simulink model "lab1"  (R2020a)
settings: Solver=VariableStepAuto  StartTime=0.0  StopTime=100  RelTol=1e-3
settings Model: Creator=L1.3-21_2  LastModifiedBy=admin
settings DataIOCC: ReturnWorkspaceOutputs=off
settings DebuggingCC: ArithmeticOperatorsInVariantConditions=warning
settings SFSimCC: SimUseLocalCustomCode=off  CustomCodeUndefinedFunction=UseInterfaceOnly
settings RTWCC: RTWUseLocalCustomCode=off

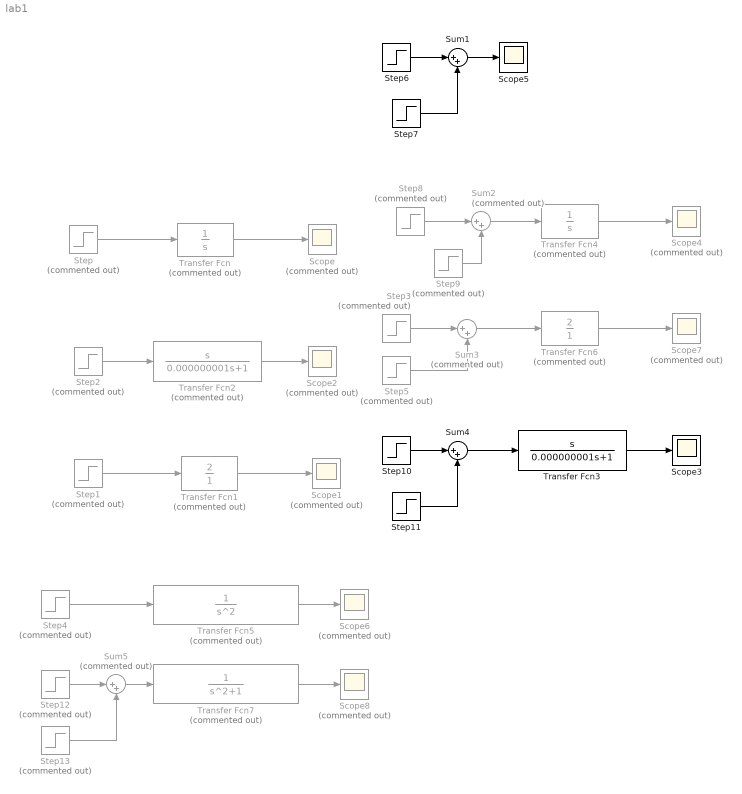
== system lab1 ==
  Scope{,1..2,4,6..8} (7 alike) : Scope  Commented=on
  Scope3 : Scope
  Scope5 : Scope
  Step{,1..2,4} (4 alike) : Step  Commented=on  SampleTime=0
  Step10 : Step  After=100000  SampleTime=0
  Step11 : Step  Time=1.0001  After=-100000  SampleTime=0
  Step12 : Step  Commented=on  After=100000  SampleTime=0
  Step13 : Step  Commented=on  Time=1.0001  After=-100000  SampleTime=0
  Step3 : Step  Commented=on  After=100000  SampleTime=0
  Step5 : Step  Commented=on  Time=1.00001  After=-100000  SampleTime=0
  Step6 : Step  After=100000  SampleTime=0
  Step7 : Step  Time=1.0001  After=-100000  SampleTime=0
  Step8 : Step  Commented=on  After=100000  SampleTime=0
  Step9 : Step  Commented=on  Time=1.00001  After=-100000  SampleTime=0
  Sum1 : Sum  Inputs=|++
  Sum2 : Sum  Commented=on  Inputs=|++
  Sum3 : Sum  Commented=on  Inputs=|++
  Sum4 : Sum  Inputs=|++
  Sum5 : Sum  Commented=on  Inputs=|++
  Transfer Fcn : TransferFcn  Commented=on  Denominator=[1 0]
  Transfer Fcn1 : TransferFcn  Commented=on  Numerator=[2]  Denominator=[1]
  Transfer Fcn2 : TransferFcn  Commented=on  Numerator=[1 0]  Denominator=[0.000000001 1]
  Transfer Fcn3 : TransferFcn  Numerator=[1 0]  Denominator=[0.000000001 1]
  Transfer Fcn4 : TransferFcn  Commented=on  Denominator=[1 0]
  Transfer Fcn5 : TransferFcn  Commented=on  Denominator=[1 0 0]
  Transfer Fcn6 : TransferFcn  Commented=on  Numerator=[2]  Denominator=[1]
  Transfer Fcn7 : TransferFcn  Commented=on  Denominator=[1 0 1]
  wires:
  Step/1 -> Transfer Fcn/1
  Transfer Fcn/1 -> Scope/1
  Transfer Fcn1/1 -> Scope1/1
  Step1/1 -> Transfer Fcn1/1
  Transfer Fcn2/1 -> Scope2/1
  Step2/1 -> Transfer Fcn2/1
  Transfer Fcn4/1 -> Scope4/1
  Step6/1 -> Sum1/1
  Step7/1 -> Sum1/2
  Sum1/1 -> Scope5/1
  Step8/1 -> Sum2/1
  Step9/1 -> Sum2/2
  Sum2/1 -> Transfer Fcn4/1
  Transfer Fcn6/1 -> Scope7/1
  Step5/1 -> Sum3/2
  Step3/1 -> Sum3/1
  Sum3/1 -> Transfer Fcn6/1
  Sum4/1 -> Transfer Fcn3/1
  Transfer Fcn3/1 -> Scope3/1
  Step10/1 -> Sum4/1
  Step11/1 -> Sum4/2
  Transfer Fcn5/1 -> Scope6/1
  Step4/1 -> Transfer Fcn5/1
  Step12/1 -> Sum5/1
  Step13/1 -> Sum5/2
  Sum5/1 -> Transfer Fcn7/1
  Transfer Fcn7/1 -> Scope8/1
